simulink model "Copy_of_ACC_GT"  (R2025b)
settings: Solver=ode4  StartTime=0  StopTime=300  FixedStep=0.001  RelTol=1e-3  EnableMultiTasking=on
libraries: Solver_SF x2
settings Model: ExtModeTrigMode=oneshot  ExtModeArmWhenConnect=off  Creator=dhall  LastModifiedBy=user
settings SolverCC: AlgebraicLoopSolver=TrustRegion  AutoInsertRateTranBlk=on
settings DataIOCC: SaveFormat=Array  SignalLoggingSaveFormat=ModelDataLogs  ReturnWorkspaceOutputs=off  SignalLoggingName=sigsOut
settings OptimizationCC: BooleanDataType=off  LocalBlockOutputs=off  InitFltsAndDblsToZero=on  LifeSpan=inf
settings DebuggingCC: SaveWithParameterizedLinksMsg=none  UnderspecifiedInitializationDetection=Classic  MergeDetectMultiDrivingBlocksExec=none  SignalResolutionControl=TryResolveAllWithWarning  MultiTaskDSMMsg=warning  MultiTaskCondExecSysMsg=none  FcnCallInpInsideContextMsg=warning  UnconnectedInputMsg=warning  UnconnectedOutputMsg=warning  UnconnectedLineMsg=warning  StateNameClashWarn=warning  SFUnexpectedBacktrackingDiag=warning  SFNoUnconditionalDefaultTransitionDiag=warning  SFExecutionAtInitializationDiag=none  ArithmeticOperatorsInVariantConditions=warning
settings HardwareCC: TargetBitPerPointer=64.0  TargetBitPerSizeT=64.0  TargetBitPerPtrDiffT=64.0  TargetLongLongMode=on  TargetIntDivRoundTo=Zero  TargetEndianess=LittleEndian  TargetWordSize=64.0  TargetPreprocMaxBitsSint=64.0  TargetPreprocMaxBitsUint=64.0  TargetHWDeviceType=MATLAB Host  ProdEqTarget=off
settings ModelReferenceCC: EnableRefExpFcnMdlSchedulingChecks=on  PropagateSignalLabelsOutOfModel=off
settings SFSimCC: SimUseLocalCustomCode=off  CustomCodeUndefinedFunction=UseInterfaceOnly
settings RTWCC: RTWUseLocalCustomCode=off  GPUComputeCapability=3.5  DLArmComputeVersion=19.05
settings CodeAppCC: StateflowObjectComments=on
settings GRTTargetCC: TargetFcnLib=ansi_tfl_tmw.mat  TargetLangStandard=C89/C90 (ANSI)  CompOptLevelCompliant=off  CombineOutputUpdateFcns=off  GRTInterface=on
settings ConfigComp: CovMetricSettings=dw  CovSaveCumulativeToWorkspaceVar=on  CovSaveSingleToWorkspaceVar=on  CovExternalEMLEnable=off

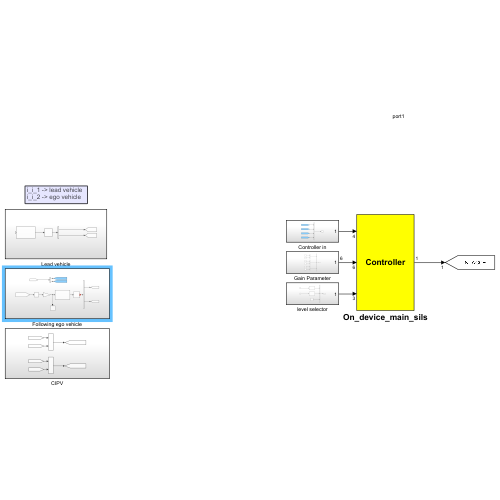
[thumbnail: Simulink's stored preview of the top-level diagram]
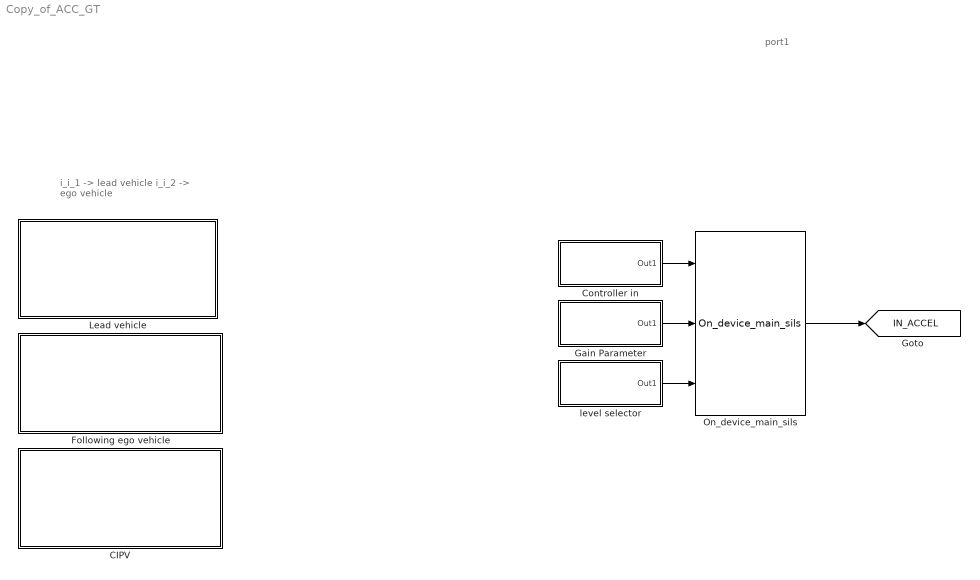
== system Copy_of_ACC_GT ==
  note: i_i_1 -> lead vehicle
      | i_i_2 -> ego vehicle
  note: port1
  CIPV : Subsystem
  Controller in : Subsystem
  Following ego vehicle : Subsystem
  Gain Parameter : Subsystem
  Lead vehicle : Subsystem
  On_device_main_sils : S-Function  FunctionName=On_device_main_sils  SFunctionDeploymentMode=off  EnableBusSupport=off
      mask Display: disp('Controller')
  level selector : Subsystem
  tag scope: IN_ACCEL=global
  wires:
  Gain Parameter/1(Out1) -> On_device_main_sils/2
  level selector/1(Out1) -> On_device_main_sils/3
  On_device_main_sils/1 -> [IN_ACCEL]
  Controller in/1(Out1) -> On_device_main_sils/1

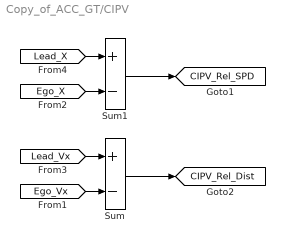
== system Copy_of_ACC_GT/CIPV ==
  Sum : Sum  Inputs=+-
  Sum1 : Sum  Inputs=+-
  tag scope: CIPV_Rel_Dist=global, CIPV_Rel_SPD=global
  wires:
  [Ego_Vx] -> Sum/2
  [Lead_Vx] -> Sum/1
  [Ego_X] -> Sum1/2
  [Lead_X] -> Sum1/1
  Sum1/1 -> [CIPV_Rel_SPD]
  Sum/1 -> [CIPV_Rel_Dist]

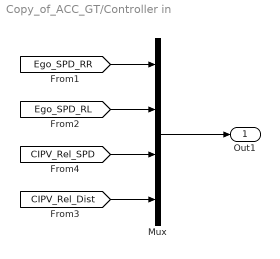
== system Copy_of_ACC_GT/Controller in ==
  Mux : Mux
  Out1 : Outport
  wires:
  Mux/1 -> Out1/1
  [Ego_SPD_RR] -> Mux/1
  [Ego_SPD_RL] -> Mux/2
  [CIPV_Rel_SPD] -> Mux/3
  [CIPV_Rel_Dist] -> Mux/4

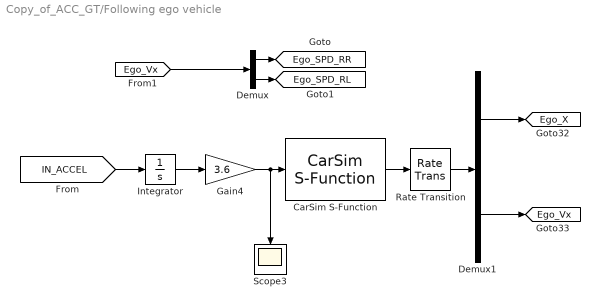
== system Copy_of_ACC_GT/Following ego vehicle ==
  CarSim S-Function : Solver_SF/CarSim S-Function  Priority=1  VehicleCode=i_i_2  SIMFILE=simfile2.sim
  Demux : Demux  Outputs=2
  Demux1 : Demux  Outputs=2
  Gain4 : Gain  Gain=3.6
  Integrator : Integrator
  Rate Transition : RateTransition  Integrity=off  OutPortSampleTime=Tc
  Scope3 : Scope
      settings: ActiveDisplayYMinimum=-113.54144428649751  ActiveDisplayYMaximum=545.2152515104674
  tag scope: Ego_SPD_RL=global, Ego_SPD_RR=global, Ego_Vx=global, Ego_X=global
  wires:
  Gain4/1 -> Scope3/1, CarSim S-Function/1
  Integrator/1 -> Gain4/1
  [IN_ACCEL] -> Integrator/1
  CarSim S-Function/1 -> Rate Transition/1
  Demux1/2 -> [Ego_Vx]
  Demux1/1 -> [Ego_X]
  Rate Transition/1 -> Demux1/1
  [Ego_Vx] -> Demux/1
  Demux/1 -> [Ego_SPD_RR]
  Demux/2 -> [Ego_SPD_RL]

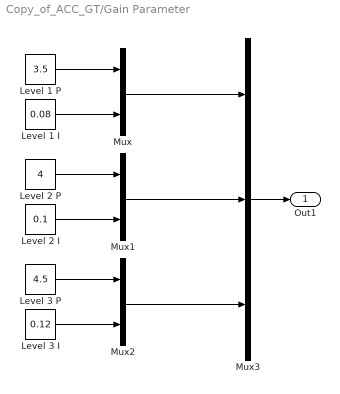
== system Copy_of_ACC_GT/Gain Parameter ==
  Level 1 I : Constant  Value=0.08
  Level 1 P : Constant  Value=3.5
  Level 2 I : Constant  Value=0.1
  Level 2 P : Constant  Value=4
  Level 3 I : Constant  Value=0.12
  Level 3 P : Constant  Value=4.5
  Mux : Mux  Inputs=2
  Mux1 : Mux  Inputs=2
  Mux2 : Mux  Inputs=2
  Mux3 : Mux  Inputs=3
  Out1 : Outport
  wires:
  Mux2/1 -> Mux3/3
  Mux/1 -> Mux3/1
  Mux1/1 -> Mux3/2
  Mux3/1 -> Out1/1
  Level 1 P/1 -> Mux/1
  Level 1 I/1 -> Mux/2
  Level 2 I/1 -> Mux1/2
  Level 2 P/1 -> Mux1/1
  Level 3 I/1 -> Mux2/2
  Level 3 P/1 -> Mux2/1

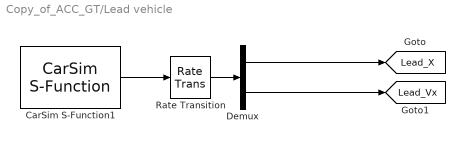
== system Copy_of_ACC_GT/Lead vehicle ==
  CarSim S-Function1 : Solver_SF/CarSim S-Function  Priority=1  VehicleCode=i_i_1  SIMFILE=simfile1.sim
  Demux : Demux  Outputs=2
  Rate Transition : RateTransition  Integrity=off  OutPortSampleTime=Tc
  tag scope: Lead_Vx=global, Lead_X=global
  wires:
  Rate Transition/1 -> Demux/1
  CarSim S-Function1/1 -> Rate Transition/1
  Demux/1 -> [Lead_X]
  Demux/2 -> [Lead_Vx]

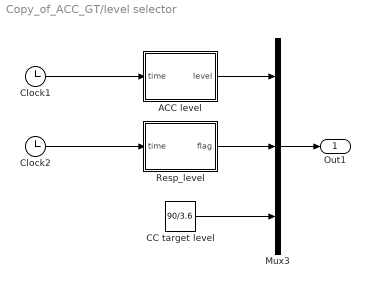
== system Copy_of_ACC_GT/level selector ==
  ACC level : MATLAB Function  TreatAsAtomicUnit=on
  CC target level : Constant  Value=90/3.6
  Clock1 : Clock
  Clock2 : Clock
  Mux3 : Mux  Inputs=3
  Resp_level : MATLAB Function  TreatAsAtomicUnit=on
  Out1 : Outport
  wires:
  Mux3/1 -> Out1/1
  Resp_level/1(flag) -> Mux3/2
  Clock2/1 -> Resp_level/1(time)
  ACC level/1(level) -> Mux3/1
  Clock1/1 -> ACC level/1(time)
  CC target level/1 -> Mux3/3

== matlab function Copy_of_ACC_GT/level selector/Resp_level ==
  data: time input; flag output
function flag = timeFlag(time)

    if time <= 0
        flag = 1;
    else
        flag = mod(ceil(time / 30) - 1, 3) + 1;
    end

end

== matlab function Copy_of_ACC_GT/level selector/ACC level ==
  data: time input; level output
function level = levelselect(time)
    if time == 0
        level = 1;
    else
        level = mod(ceil(time / 90) - 1, 3) + 1;
    end
end
